simulink model "Parameter_estimation"  (R2025b)
settings: Solver=VariableStepAuto  StartTime=0.0  StopTime=25000  FixedStep=1
libraries: fl_lib x11, nesl_utility x11, batt_lib x6, ee_lib x1
settings Model: Creator=faxio  LastModifiedBy=faxio

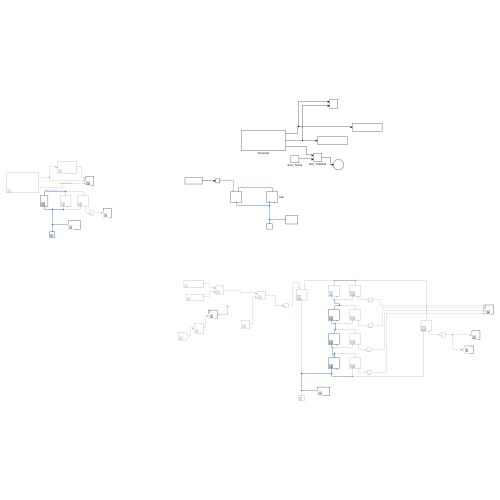
[thumbnail: Simulink's stored preview of the top-level diagram]
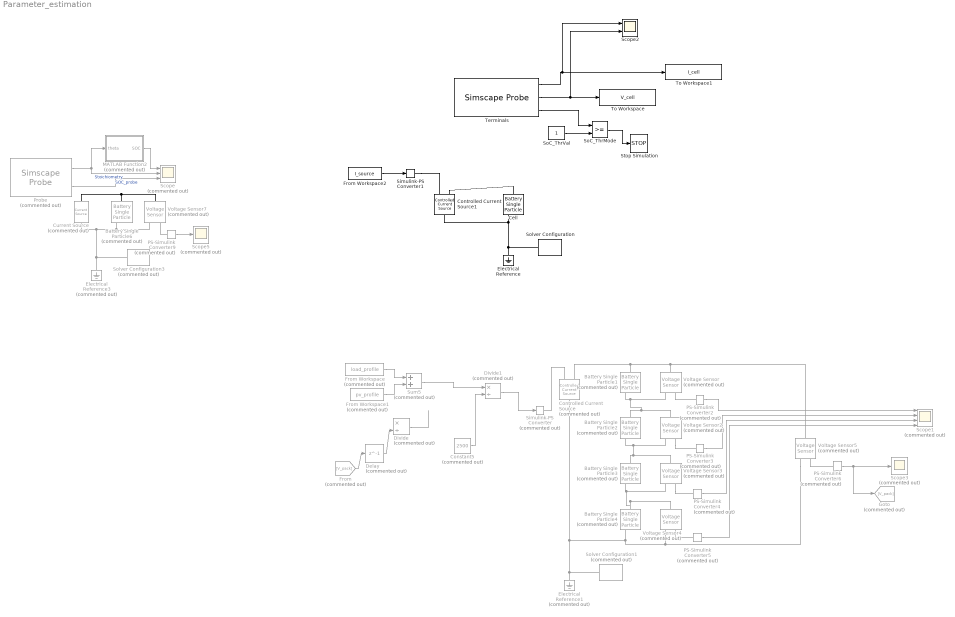
== system Parameter_estimation ==
  Battery Single Particle{1..4,6} (5 alike) : batt_lib/Cells/Electrochemical/Battery Single Particle  Commented=on  ExtrapolationMethod=simscape.enum.extrapolation.nearest  ThicknessAnode=3.4E-5 m  ElectrolyteLayerCountAnode=10  ThicknessSeparator=2.5E-5 m  ElectrolyteLayerCountSeparator=5  ThicknessCathode=8E-5 m  ElectrolyteLayerCountCathode=10  ElectrodePlateArea=1.8E-1 m^2  ParticleRadiusAnode=5E-6 m  ShellCountAnode=10  ParticleRadiusCathode=5E-8 m  ShellCountCathode=10  ActiveMaterialVolumeFractionAnode=0.58  ActiveMaterialVolumeFractionCathode=0.374  StoichiometryBreakpointsSpecification=simscape.battery.enum.cells.electrochemical.StoichiometryBreakpointsSpecification.normalized  NormalizedStoichiometryBreakpoints=linspace(0.025, 0.975, 39)  OpenCircuitPotentialAnode=[.435; .325; .259; .221; .204; .194; .179; .166; .155; .145; .137; .131; .128; .127; .126; .125; .124; .123; .122; .121; .118; .117; .112; .109; .105; .1; .098; .095; .094; .093; .091; .09; .089; .088; .087; .086; .085; .084; .083] V  OpenCircuitPotentialCathode=[3.598; 3.53; 3.494; 3.474; 3.46; 3.455; 3.454; 3.453; 3.4528; 3.4526; 3.4524; 3.452; 3.4518; 3.4516; 3.4514; 3.4512; 3.451; 3.4508; 3.4506; 3.4503; 3.45; 3.4498; 3.4495; 3.4493; 3.449; 3.4488; 3.4486; 3.4484; 3.4482; 3.4479; 3.4477; 3.4475; 3.4473; 3.447; 3.4468; 3.4466; 3.4464; 3.4462; 3.4458] V  AbsoluteStoichiometryBreakpointsAnode=linspace(0.025, 0.975, 39)  OpenCircuitPotentialAbsoluteAnode=[.484; .335; .253; .209; .2; .181; .165; .151; .139; .131; .128; .125; .124; .124; .123; .122; .119; .117; .111; .108; .101; .098; .095; .093; .092; .088; .088; .088; .088; .087; .087; .087; .085; .082; .079; .071; .064; .049; .026] V  AbsoluteStoichiometryBreakpointsCathode=linspace(0.025, 0.975, 39)  OpenCircuitPotentialAbsoluteCathode=[3.81; 3.608; 3.512; 3.478; 3.459; 3.453; 3.45257; 3.45214; 3.45171; 3.45128; 3.45085; 3.45042; 3.44999; 3.44956; 3.44913; 3.4487; 3.44827; 3.44784; 3.44741; 3.44698; 3.44655; 3.44612; 3.44569; 3.44526; 3.44483; 3.4444; 3.44397; 3.44354; 3.44311; 3.44268; 3.44225; 3.44182; 3.44139; 3.44096; 3.44053; 3.44; 3.412; 3.304; 2.968] V  MaximumConcentrationAnode=30555 mol/m^3  MaximumStoichiometryAnode=0.811  MinimumStoichiometryAnode=0.0132  MaximumConcentrationCathode=22806 mol/m^3  MaximumStoichiometryCathode=0.74  MinimumStoichiometryCathode=0.035  ActiveMaterialDiffusionCoefficientAnode=3E-15 m^2/s  ActiveMaterialDiffusionCoefficientCathode=5.9E-20 m^2/s  ConductivityAnode=100 S/m  ConductivityCathode=0.5 S/m  CurrentCollectorResistance=0 Ohm  ElectrolyteVolumeFractionAnode=0.3874  ElectrolyteVolumeFractionSeparator=0.45  ElectrolyteVolumeFractionCathode=0.5725  ElectrolyteConductivity=0.29 S/m  BruggemanExponentAnode=1.5  BruggemanExponentSeparator=1.5  BruggemanExponentCathode=1.5  TransferenceNumber=0.363  ElectrolyteDiffusionCoefficient=2E-10 m^2/s  ChargeTransferRateAnode=8.8E-11 m^(5/2)/(mol^(1/2)*s)  ChargeTransferRateCathode=2.8E-13 m^(5/2)/(mol^(1/2)*s)  BatteryThermalMass=77 J/K  ArrheniusReferenceTemperature=298.15 K  ActiveMaterialDiffusionActivationEnergyAnode=39000 J/mol  ActiveMaterialDiffusionActivationEnergyCathode=35000 J/mol  ElectrolyteDiffusionActivationEnergy=26600 J/mol  ConductivityActivationEnergyAnode=3000 J/mol  ConductivityActivationEnergyCathode=3000 J/mol  ElectrolyteConductivityActivationEnergy=11000 J/mol  ChargeTransferActivationEnergyAnode=13000 J/mol  ChargeTransferActivationEnergyCathode=20000 J/mol  batteryCurrent_specify=off  batteryCurrent_priority=None  batteryCurrent=0 A  batteryCurrent_nominal_specify=off  batteryCurrent_nominal_value=1  batteryCurrent_nominal_unit=A  batteryVoltage_specify=off  batteryVoltage_priority=None  batteryVoltage=0 V  batteryVoltage_nominal_specify=off  batteryVoltage_nominal_value=1  batteryVoltage_nominal_unit=V  averageElectrolyteConcentration_specify=off  averageElectrolyteConcentration_priority=High  averageElectrolyteConcentration=1200 mol/m^3  averageElectrolyteConcentration_nominal_specify=off  averageElectrolyteConcentration_nominal_value=1  averageElectrolyteConcentration_nominal_unit=mol/m^3  stateOfCharge_specify=on  stateOfCharge_priority=High  stateOfCharge=1  stateOfCharge_nominal_specify=off  stateOfCharge_nominal_value=1  stateOfCharge_nominal_unit=1  batteryTemperature_specify=off  batteryTemperature_priority=High  batteryTemperature=298.15 K  batteryTemperature_nominal_specify=off  batteryTemperature_nominal_value=1  batteryTemperature_nominal_unit=K  power_dissipated_specify=off  power_dissipated_priority=None  power_dissipated=0 W  power_dissipated_nominal_specify=off  power_dissipated_nominal_value=1  power_dissipated_nominal_unit=W  heatGenerationRate_specify=off  heatGenerationRate_priority=None  heatGenerationRate=0 W  heatGenerationRate_nominal_specify=off  heatGenerationRate_nominal_value=1  heatGenerationRate_nominal_unit=W
      settings: InternalSimscapePortConfiguration="{\"Bottom\":[],\"Left\":[{\"id\":\"p\",\"label\":\"+\",\"type\":\"foundation.electrical.electrical\"}],\"Right\":[{\"id\":\"n\",\"label\":\"-\",\"type\":\"foundation.electrical.electrical\"},{\"id\":\"H\",\"label\":\"H\",\"type\":\"foundation.thermal.thermal\"}],\"Top\":[]}"
  Cell : batt_lib/Cells/Electrochemical/Battery Single Particle  ExtrapolationMethod=simscape.enum.extrapolation.nearest  ThicknessAnode=0.000147 m  ElectrolyteLayerCountAnode=10  ThicknessSeparator=2.5e-05 m  ElectrolyteLayerCountSeparator=5  ThicknessCathode=0.0001 m  ElectrolyteLayerCountCathode=10  ElectrodePlateArea=1 m^2  ParticleRadiusAnode=1.2e-05 m  ShellCountAnode=10  ParticleRadiusCathode=5e-06 m  ShellCountCathode=10  ActiveMaterialVolumeFractionAnode=0.466  ActiveMaterialVolumeFractionCathode=0.49  StoichiometryBreakpointsSpecification=simscape.battery.enum.cells.electrochemical.StoichiometryBreakpointsSpecification.normalized  NormalizedStoichiometryBreakpoints=[0 0.0101010101010101 0.0202020202020202 0.0303030303030303 0.0404040404040404 0.0505050505050505 0.0606060606060606 0.0707070707070707 0.0808080808080808 0.0909090909090909 0.101010101010101 0.111111111111111 0.121212121212121 0.131313131313131 0.141414141414141 0.151515151515152 0.161616161616162 0.171717171717172 0.181818181818182 0.191919191919192 0.202020202020202 0.212121212121212 0.222222222222222 0.232323232323232 0.242424242424242 0.252525252525253 0.262626262626263 0.272727272727273 0.282828282828283 0.292929292929293 0.303030303030303 0.313131313131313 0.323232323232323 0.333333333333333 0.343434343434343 0.353535353535354 0.363636363636364 0.373737373737374 0.383838383838384 0.393939393939394 0.404040404040404 0.414141414141414 0.424242424242424 0.434343434343434 0.444444444444444 0.454545454545455 0.464646464646465 0.474747474747475 0.484848484848485 0.494949494949495 0.505050505050505 0.515151515151515 0.525252525252525 0.535353535353535 0.545454545454545 0.555555555555556 0.565656565656566 0.575757575757576 0.585858585858586 0.595959595959596 0.606060606060606 0.616161616161616 0.626262626262626 0.636363636363636 0.646464646464647 0.656565656565657 0.666666666666667 0.676767676767677 0.686868686868687 0.696969696969697 0.707070707070707 0.717171717171717 0.727272727272727 0.737373737373737 0.747474747474748 0.757575757575758 0.767676767676768 0.777777777777778 0.787878787878788 0.797979797979798 0.808080808080808 0.818181818181818 0.828282828282828 0.838383838383838 0.848484848484849 0.858585858585859 0.868686868686869 0.878787878787879 0.888888888888889 0.898989898989899 0.909090909090909 0.919191919191919 0.929292929292929 0.939393939393939 0.94949494949495 0.95959595959596 0.96969696969697 0.97979797979798 0.98989898989899 1]  OpenCircuitPotentialAnode=[0.527805774432301 0.389705202310941 0.316765913197973 0.277734911673862 0.256581346925095 0.244922969374972 0.238340163681284 0.234487508773189 0.232107919789912 0.230509810044929 0.229278173973024 0.228089643344467 0.226541418665581 0.223926190789775 0.219033051764386 0.210667406696483 0.199675061560496 0.189227936899446 0.1809519745655 0.174002446195912 0.167319751949806 0.160633694230646 0.154273713587729 0.148713222459875 0.144236467425281 0.140852488610362 0.138383876420472 0.136590425081163 0.135250629454596 0.134195687269057 0.133316625227257 0.132561672963033 0.131930558712017 0.13146436845018 0.131227066498425 0.131279136591051 0.131652071638428 0.132335773102896 0.133283598353663 0.134428346836364 0.135697878759629 0.137022977691537 0.138335903362948 0.139560633629842 0.140594285300427 0.141273715047302 0.141309702154789 0.140156165958355 0.136829939365833 0.130096960211683 0.120098063408118 0.110014499158857 0.103025424247891 0.0992349196487724 0.0973781349307678 0.0964948544583568 0.0960970194192093 0.0959591085852174 0.095973451976035 0.0960837617826242 0.0962574947293819 0.0964742716749206 0.0967206671882491 0.0969875910359484 0.0972688081570556 0.0975600196830932 0.0978582571609871 0.0981614703027366 0.0984682422830865 0.0987775919206351 0.099088835774949 0.0994014915213533 0.0997152093993002 0.100029722156565 0.100344806271279 0.100660248617054 0.100975813283391 0.101291202993936 0.101606008375021 0.101919635962317 0.102231201838676 0.102539371429581 0.102842116084738 0.103136341872894 0.103417322845859 0.10367783594507 0.103906842043959 0.104087479464262 0.10419402254355 0.104187297399709 0.104007833097212 0.103565771014671 0.102726325436733 0.101289586829772 0.0989641829612105 0.095336811474051 0.0898457748126877 0.0817786360773103 0.0703318537979337 0.0547833971431165] V  OpenCircuitPotentialCathode=[4.2550850722288 4.23964234870498 4.22473702607522 4.2103336684674 4.19640053146682 4.18290905449932 4.16983343847436 4.15715029196502 4.14483833292082 4.13287813570988 4.1212519154173 4.10994334296204 4.09893738586109 4.0882201704585 4.07777886221477 4.06760156126839 4.05767721097313 4.04799551750946 4.03854687898709 4.02932232271497 4.02031344952625 4.01151238421969 4.00291173132193 3.99450453549408 3.98628424600448 3.97824468477258 3.97038001755795 3.96268472792673 3.95515359367772 3.94778166545159 3.94056424728312 3.93349687888619 3.92657531948797 3.91979553305088 3.91315367474036 3.90664607851333 3.9002692457167 3.89401983459771 3.88789465063926 3.8818906376427 3.87600486948899 3.87023454251661 3.86457696846107 3.85902956790649 3.85358986420482 3.84825547782287 3.84302412108089 3.83789359325051 3.83286177598237 3.82792662903711 3.82308618629542 3.81833855202541 3.81368189738731 3.80911445715743 3.80463452665491 3.80024045885615 3.79593066168318 3.79170359545333 3.78755777047883 3.78349174480548 3.779504122081 3.77559354954393 3.77175871612491 3.76799835065286 3.76431122015905 3.76069612827253 3.75715191370123 3.75367744879295 3.7502716381714 3.74693341744244 3.74366175196622 3.7404556356911 3.73731409004562 3.73423616288467 3.73122092748635 3.72826748159485 3.72537494650286 3.72254246616031 3.71976920627804 3.71705435334527 3.71439711334181 3.71179670954953 3.70925237783427 3.70676335493894 3.70432884757156 3.70194794881732 3.69961941016288 3.69734101783265 3.69510788484459 3.69290777195411 3.69070826732289 3.68842165799218 3.68580867394662 3.68221473504698 3.67584723388283 3.66179519698305 3.62660289820017 3.53340085028017 3.28116277753662 2.59306439239881] V  AbsoluteStoichiometryBreakpointsAnode=linspace(0.025, 0.975, 39)  OpenCircuitPotentialAbsoluteAnode=[.484; .335; .253; .209; .2; .181; .165; .151; .139; .131; .128; .125; .124; .124; .123; .122; .119; .117; .111; .108; .101; .098; .095; .093; .092; .088; .088; .088; .088; .087; .087; .087; .085; .082; .079; .071; .064; .049; .026] V  AbsoluteStoichiometryBreakpointsCathode=linspace(0.025, 0.975, 39)  OpenCircuitPotentialAbsoluteCathode=[3.81; 3.608; 3.512; 3.478; 3.459; 3.453; 3.45257; 3.45214; 3.45171; 3.45128; 3.45085; 3.45042; 3.44999; 3.44956; 3.44913; 3.4487; 3.44827; 3.44784; 3.44741; 3.44698; 3.44655; 3.44612; 3.44569; 3.44526; 3.44483; 3.4444; 3.44397; 3.44354; 3.44311; 3.44268; 3.44225; 3.44182; 3.44139; 3.44096; 3.44053; 3.44; 3.412; 3.304; 2.968] V  MaximumConcentrationAnode=31850 mol/m^3  MaximumStoichiometryAnode=0.97  MinimumStoichiometryAnode=0.02  MaximumConcentrationCathode=52500 mol/m^3  MaximumStoichiometryCathode=0.99  MinimumStoichiometryCathode=0.19  ActiveMaterialDiffusionCoefficientAnode=2.7814e-13 m^2/s  ActiveMaterialDiffusionCoefficientCathode=1.67e-14 m^2/s  ConductivityAnode=100 S/m  ConductivityCathode=0.5 S/m  CurrentCollectorResistance=4.4948e-08 Ohm  ElectrolyteVolumeFractionAnode=0.477  ElectrolyteVolumeFractionSeparator=0.45  ElectrolyteVolumeFractionCathode=0.36  ElectrolyteConductivity=1.17 S/m  BruggemanExponentAnode=1.86  BruggemanExponentSeparator=1.5  BruggemanExponentCathode=2.26  TransferenceNumber=0.38  ElectrolyteDiffusionCoefficient=2.811e-10 m^2/s  ChargeTransferRateAnode=8.8E-11 m^(5/2)/(mol^(1/2)*s)  ChargeTransferRateCathode=2.8E-13 m^(5/2)/(mol^(1/2)*s)  BatteryThermalMass=77 J/K  ArrheniusReferenceTemperature=298.15 K  ActiveMaterialDiffusionActivationEnergyAnode=50000 J/mol  ActiveMaterialDiffusionActivationEnergyCathode=25000 J/mol  ElectrolyteDiffusionActivationEnergy=26600 J/mol  ConductivityActivationEnergyAnode=3000 J/mol  ConductivityActivationEnergyCathode=3000 J/mol  ElectrolyteConductivityActivationEnergy=11000 J/mol  ChargeTransferActivationEnergyAnode=30000 J/mol  ChargeTransferActivationEnergyCathode=30000 J/mol  batteryCurrent_specify=off  batteryCurrent_priority=None  batteryCurrent=0 A  batteryCurrent_nominal_specify=off  batteryCurrent_nominal_value=1  batteryCurrent_nominal_unit=A  batteryVoltage_specify=off  batteryVoltage_priority=None  batteryVoltage=0 V  batteryVoltage_nominal_specify=off  batteryVoltage_nominal_value=1  batteryVoltage_nominal_unit=V  averageElectrolyteConcentration_specify=off  averageElectrolyteConcentration_priority=High  averageElectrolyteConcentration=1200 mol/m^3  averageElectrolyteConcentration_nominal_specify=off  averageElectrolyteConcentration_nominal_value=1  averageElectrolyteConcentration_nominal_unit=mol/m^3  stateOfCharge_specify=on  stateOfCharge_priority=High  stateOfCharge=0  stateOfCharge_nominal_specify=off  stateOfCharge_nominal_value=1  stateOfCharge_nominal_unit=1  batteryTemperature_specify=off  batteryTemperature_priority=High  batteryTemperature=298.15 K  batteryTemperature_nominal_specify=off  batteryTemperature_nominal_value=1  batteryTemperature_nominal_unit=K  power_dissipated_specify=off  power_dissipated_priority=None  power_dissipated=0 W  power_dissipated_nominal_specify=off  power_dissipated_nominal_value=1  power_dissipated_nominal_unit=W  heatGenerationRate_specify=off  heatGenerationRate_priority=None  heatGenerationRate=0 W  heatGenerationRate_nominal_specify=off  heatGenerationRate_nominal_value=1  heatGenerationRate_nominal_unit=W
      settings: InternalSimscapePortConfiguration="{\"Bottom\":[],\"Left\":[{\"id\":\"p\",\"label\":\"+\",\"type\":\"foundation.electrical.electrical\"}],\"Right\":[{\"id\":\"n\",\"label\":\"-\",\"type\":\"foundation.electrical.electrical\"},{\"id\":\"H\",\"label\":\"H\",\"type\":\"foundation.thermal.thermal\"}],\"Top\":[]}"
  Constant5 : Constant  Commented=on  Value=2500
  Controlled Current Source : fl_lib/Electrical/Electrical Sources/Controlled Current Source  Commented=on
  Controlled Current Source1 : fl_lib/Electrical/Electrical Sources/Controlled Current Source
  Current Source : ee_lib/Sources/Current Source  Commented=on  dc_current=1 A  ac_current=0 A  ac_shift=0 rad  ac_frequency=60 Hz  noise_mode=ee.enum.sources.noise.Disabled  PSD=0 A^2/Hz  sample_time=1e-3 s  repeatability=ee.enum.sources.repeatability.NotRepeatable  user_seed=0  auto_seed=545404223  i_specify=off  i_priority=None  i=0 A  i_nominal_specify=off  i_nominal_value=1  i_nominal_unit=A  v_specify=off  v_priority=None  v=0 V  v_nominal_specify=off  v_nominal_value=1  v_nominal_unit=V
  Delay : Delay  Commented=on  DelayLength=1  InputProcessing=Columns as channels (frame based)
  Divide : Product  Commented=on  Inputs=*/
  Divide1 : Product  Commented=on  Inputs=*/
  Electrical Reference : fl_lib/Electrical/Electrical Elements/Electrical Reference
  Electrical Reference1 : fl_lib/Electrical/Electrical Elements/Electrical Reference  Commented=on
  Electrical Reference3 : fl_lib/Electrical/Electrical Elements/Electrical Reference  Commented=on
  From : From  Commented=on  GotoTag=V_pack
  From Workspace : FromWorkspace  Commented=on  VariableName=load_profile
  From Workspace1 : FromWorkspace  Commented=on  VariableName=pv_profile
  From Workspace2 : FromWorkspace  VariableName=I_source
  Goto : Goto  Commented=on  GotoTag=V_pack
  MATLAB Function2 : MATLAB Function  Commented=on  TreatAsAtomicUnit=on
  PS-Simulink Converter{2..6,9} (6 alike) : nesl_utility/PS-Simulink Converter  Commented=on  PhysicalDomain=network_engine_domain  SubClassName=ps_output  LeftPortType=input  RightPortType=output  PseudoPeriodic=off  Frequencies=[]  VectorFormat=inherit  Unit=inherit  AffineConversion=off
  Probe : SimscapeProbe  Commented=on  BoundBlock=104  Variables="{\"anodeModel.averageStoichiometry\":{\"Probing\":\"ON\"},\"stateOfCharge\":{\"Probing\":\"ON\"}}"
  Scope : Scope  Commented=on  NumInputPorts=3
      settings: ActiveDisplayYMinimum=-0.0847899241822074  ActiveDisplayYMaximum=1.1205322137980231  DataLoggingVariableName=ScopeData5
  Scope1 : Scope  Commented=on  NumInputPorts=4
      settings: ActiveDisplayYMinimum=-1  ActiveDisplayYMaximum=1
  Scope2 : Scope  NumInputPorts=2
      settings: ActiveDisplayYMinimum=-6.9799999999999986  ActiveDisplayYMaximum=62.820000000000007  DataLoggingVariableName=ScopeData2
  Scope3 : Scope  Commented=on
      settings: ActiveDisplayYMinimum=11.851885488512112  ActiveDisplayYMaximum=13.610571697723437  DataLoggingVariableName=ScopeData3
  Scope5 : Scope  Commented=on
      settings: ActiveDisplayYMinimum=2.8486897054184919  ActiveDisplayYMaximum=3.5597839817126782  DataLoggingVariableName=ScopeData4
  Simulink-PS Converter : nesl_utility/Simulink-PS Converter  Commented=on  PhysicalDomain=network_engine_domain  SubClassName=ps_input  LeftPortType=input  RightPortType=output  PseudoPeriodic=off  Frequencies=[]  NoiseDistribution=none  NoiseParameters=[]  Unit=1  AffineConversion=off  FilteringAndDerivatives=provide  SimscapeFilterOrder=1  InputFilterTimeConstant=0.001  UdotUserProvided=0
  Simulink-PS Converter1 : nesl_utility/Simulink-PS Converter  PhysicalDomain=network_engine_domain  SubClassName=ps_input  LeftPortType=input  RightPortType=output  PseudoPeriodic=off  Frequencies=[]  NoiseDistribution=none  NoiseParameters=[]  Unit=1  AffineConversion=off  FilteringAndDerivatives=provide  SimscapeFilterOrder=1  InputFilterTimeConstant=0.001  UdotUserProvided=0
  SoC_ThrMode : RelationalOperator  OutDataTypeStr=boolean  RndMeth=Simplest  InputSameDT=off
  SoC_ThrVal : Constant
  Solver Configuration : nesl_utility/Solver Configuration  PhysicalDomain=network_engine_domain  SubClassName=solver  LeftPortType=input  RightPortType=generic  Tones=[]  Harmonics=[]  SimulateNoise=off  Profile=off  UseLocalSampling=off  EnableSwitchedLinearOptims=on  FrequencyDomain=off  UseCCode=off  RelTol=0.001  AbsTol=0.001  MinStep=1e-09  ToWorkspace=off  RevertToSquareIcSolve=off  NumHomotopyIterations=100  PhasorMode=off  PhasorModeNumHarmonics=1  ConsistencySolver=NEWTON_XTOL_AFTER_FTOL  IndexReductionMethod=DerivativeReplacement  DoDC=off  ResidualTolerance=1e-09  ConsistencyTolSource=GLOBAL  ConsistencyAbsTol=0.001  ConsistencyRelTol=0.001  ConsistencyTolFactor=0.001  UseLocalSolver=off  LocalSolverChoice=NE_BACKWARD_EULER_ADVANCER  ResolveIndetEquations=on  FunctionEvalNumThread=1  LocalSolverSampleTime=0.001  DoFixedCost=off  MaxNonlinIter=3  MaxModeIter=2  ComputeImpulses=off  ImpulseIterations=2  LinearAlgebra=auto  LinearAlgebraNumThread=0  EquationFormulation=NE_TIME_EF  DelaysMemoryBudget=1024  AutomaticFiltering=on  FilteringTimeConstant=0.001  PartitionStorageMethod=AS_NEEDED  PartitionMemoryBudget=1024  PartitionMethod=ROBUST  MultibodyUseLocalSolver=off  MultibodyLocalSolverChoice=ODE1  MultibodyLocalSolverSampleTime=0.001
  Solver Configuration1 : nesl_utility/Solver Configuration  Commented=on  PhysicalDomain=network_engine_domain  SubClassName=solver  LeftPortType=input  RightPortType=generic  Tones=[]  Harmonics=[]  SimulateNoise=off  Profile=off  UseLocalSampling=off  EnableSwitchedLinearOptims=on  FrequencyDomain=off  UseCCode=off  RelTol=0.001  AbsTol=0.001  MinStep=1e-09  ToWorkspace=off  RevertToSquareIcSolve=off  NumHomotopyIterations=100  PhasorMode=off  PhasorModeNumHarmonics=1  ConsistencySolver=NEWTON_XTOL_AFTER_FTOL  IndexReductionMethod=DerivativeReplacement  DoDC=off  ResidualTolerance=1e-09  ConsistencyTolSource=GLOBAL  ConsistencyAbsTol=0.001  ConsistencyRelTol=0.001  ConsistencyTolFactor=0.001  UseLocalSolver=off  LocalSolverChoice=NE_BACKWARD_EULER_ADVANCER  ResolveIndetEquations=on  FunctionEvalNumThread=1  LocalSolverSampleTime=0.001  DoFixedCost=off  MaxNonlinIter=3  MaxModeIter=2  ComputeImpulses=off  ImpulseIterations=2  LinearAlgebra=auto  LinearAlgebraNumThread=0  EquationFormulation=NE_TIME_EF  DelaysMemoryBudget=1024  AutomaticFiltering=on  FilteringTimeConstant=0.001  PartitionStorageMethod=AS_NEEDED  PartitionMemoryBudget=1024  PartitionMethod=ROBUST  MultibodyUseLocalSolver=off  MultibodyLocalSolverChoice=ODE1  MultibodyLocalSolverSampleTime=0.001
  Solver Configuration3 : nesl_utility/Solver Configuration  Commented=on  PhysicalDomain=network_engine_domain  SubClassName=solver  LeftPortType=input  RightPortType=generic  Tones=[]  Harmonics=[]  SimulateNoise=off  Profile=off  UseLocalSampling=off  EnableSwitchedLinearOptims=on  FrequencyDomain=off  UseCCode=off  RelTol=0.001  AbsTol=0.001  MinStep=1e-09  ToWorkspace=off  RevertToSquareIcSolve=off  NumHomotopyIterations=100  PhasorMode=off  PhasorModeNumHarmonics=1  ConsistencySolver=NEWTON_XTOL_AFTER_FTOL  IndexReductionMethod=DerivativeReplacement  DoDC=off  ResidualTolerance=1e-09  ConsistencyTolSource=GLOBAL  ConsistencyAbsTol=0.001  ConsistencyRelTol=0.001  ConsistencyTolFactor=0.001  UseLocalSolver=off  LocalSolverChoice=NE_BACKWARD_EULER_ADVANCER  ResolveIndetEquations=on  FunctionEvalNumThread=1  LocalSolverSampleTime=0.001  DoFixedCost=off  MaxNonlinIter=3  MaxModeIter=2  ComputeImpulses=off  ImpulseIterations=2  LinearAlgebra=auto  LinearAlgebraNumThread=0  EquationFormulation=NE_TIME_EF  DelaysMemoryBudget=1024  AutomaticFiltering=on  FilteringTimeConstant=0.001  PartitionStorageMethod=AS_NEEDED  PartitionMemoryBudget=1024  PartitionMethod=ROBUST  MultibodyUseLocalSolver=off  MultibodyLocalSolverChoice=ODE1  MultibodyLocalSolverSampleTime=0.001
  Stop Simulation : Stop
  Sum5 : Sum  Commented=on
  Terminals : SimscapeProbe  BoundBlock=1  Variables="{\"batteryCurrent\":{\"Probing\":\"ON\"},\"batteryTemperature\":{\"Probing\":\"OFF\"},\"batteryVoltage\":{\"Probing\":\"ON\"},\"stateOfCharge\":{\"Probing\":\"ON\"}}"
  To Workspace : ToWorkspace  VariableName=V_cell  SaveFormat=Timeseries  SampleTime=1
  To Workspace1 : ToWorkspace  VariableName=I_cell  SaveFormat=Timeseries  SampleTime=1
  Voltage Sensor{,2..5,7} (6 alike) : fl_lib/Electrical/Electrical Sensors/Voltage Sensor  Commented=on
  wires:
  Divide1/1 -> Simulink-PS Converter/1
  Constant5/1 -> Divide1/2
  From Workspace/1 -> Sum5/1
  From Workspace1/1 -> Sum5/2
  PS-Simulink Converter2/1 -> Scope1/1
  PS-Simulink Converter3/1 -> Scope1/2
  PS-Simulink Converter4/1 -> Scope1/3
  PS-Simulink Converter5/1 -> Scope1/4
  PS-Simulink Converter6/1 -> Goto/1, Scope3/1
  From/1 -> Delay/1
  Delay/1 -> Divide/2
  Sum5/1 -> Divide1/1
  Divide/1 -> ?
  PS-Simulink Converter9/1 -> Scope5/1
  Probe/1 -> MATLAB Function2/1(theta), Scope/2  "Stoichiometry"
  Probe/2 -> Scope/3  "SOC_probe"
  MATLAB Function2/1(SOC) -> Scope/1
  Terminals/2 -> Scope2/2, To Workspace/1
  SoC_ThrVal/1 -> SoC_ThrMode/2
  SoC_ThrMode/1 -> Stop Simulation/1
  Terminals/3 -> SoC_ThrMode/1
  Terminals/1 -> To Workspace1/1, Scope2/1
  From Workspace2/1 -> Simulink-PS Converter1/1
  connections:
  Cell/LConn1 -- Controlled Current Source1/RConn2
  Cell/RConn1 -- Controlled Current Source1/LConn1 -- Electrical Reference/LConn1 -- Solver Configuration/RConn1
  Battery Single Particle2/LConn1 -- Voltage Sensor/RConn2 -- Battery Single Particle1/RConn1 -- Voltage Sensor2/LConn1
  Battery Single Particle1/LConn1 -- Controlled Current Source/RConn2 -- Voltage Sensor5/LConn1 -- Voltage Sensor/LConn1
  Simulink-PS Converter/RConn1 -- Controlled Current Source/RConn1
  Solver Configuration1/RConn1 -- Electrical Reference1/LConn1 -- Controlled Current Source/LConn1 -- Voltage Sensor4/RConn2 -- Voltage Sensor5/RConn2 -- Battery Single Particle4/RConn1
  Voltage Sensor3/RConn2 -- Battery Single Particle4/LConn1 -- Voltage Sensor4/LConn1 -- Battery Single Particle3/RConn1
  Voltage Sensor2/RConn2 -- Battery Single Particle3/LConn1 -- Voltage Sensor3/LConn1 -- Battery Single Particle2/RConn1
  Voltage Sensor/RConn1 -- PS-Simulink Converter2/LConn1
  Voltage Sensor2/RConn1 -- PS-Simulink Converter3/LConn1
  Voltage Sensor3/RConn1 -- PS-Simulink Converter4/LConn1
  Voltage Sensor4/RConn1 -- PS-Simulink Converter5/LConn1
  Voltage Sensor5/RConn1 -- PS-Simulink Converter6/LConn1
  Solver Configuration3/RConn1 -- Electrical Reference3/LConn1 -- Current Source/LConn1 -- Voltage Sensor7/RConn2 -- Battery Single Particle6/RConn1
  Battery Single Particle6/LConn1 -- Current Source/RConn1 -- Voltage Sensor7/LConn1
  PS-Simulink Converter9/LConn1 -- Voltage Sensor7/RConn1
  Simulink-PS Converter1/RConn1 -- Controlled Current Source1/RConn1

== matlab function Parameter_estimation/MATLAB Function2 ==
  data: theta input; SOC output
function SOC = fcn(theta)
theta_max=0.811;
theta_min=0.0132;

SOC= (theta-theta_min)/(theta_max-theta_min);
